simulink model "testSerializedParams"  (R2014a)
settings: Solver=FixedStepDiscrete  StartTime=0.0  StopTime=Inf  FixedStep=0.001  RelTol=1e-3
InitFcn:
  | testSerializedParams_Initialize();
undefined symbols (not defined in the file or in its folder): fn5, libBusSerialize, TestBus_serializedParam
libraries: slrtlib x5, dspswit3 x2, libButtons x1
settings Model: BufferReuse=off  Creator=shenoylab  LastModifiedBy=djoshea
settings SolverCC: EnableConcurrentExecution=on
settings DataIOCC: SignalLoggingSaveFormat=ModelDataLogs
settings OptimizationCC: BlockReduction=off  OptimizeBlockIOStorage=off  BufferReuse=off  GlobalBufferReuse=off  ExpressionFolding=off  LocalBlockOutputs=off
settings DebuggingCC: MultiTaskDSMMsg=warning  MultiTaskCondExecSysMsg=none  StateNameClashWarn=warning
settings HardwareCC: ProdIntDivRoundTo=Zero  ProdEndianess=LittleEndian  ProdHWDeviceType=Generic->32-bit x86 compatible
settings RTWCC: SystemTargetFile=slrt.tlc  TemplateMakefile=slrt_default_tmf  Description=Simulink Real-Time  GenerateReport=on  ProcessScript=slrt_make_rtw_hook  LaunchReport=on  IncludeERTFirstTime=on  RTWCompilerOptimization=On
settings CodeAppCC: MATLABSourceComments=on
settings SimulinkRealTimeCC: GeneratePreprocessorConditionals=Disable all  EnableShiftOperators=on

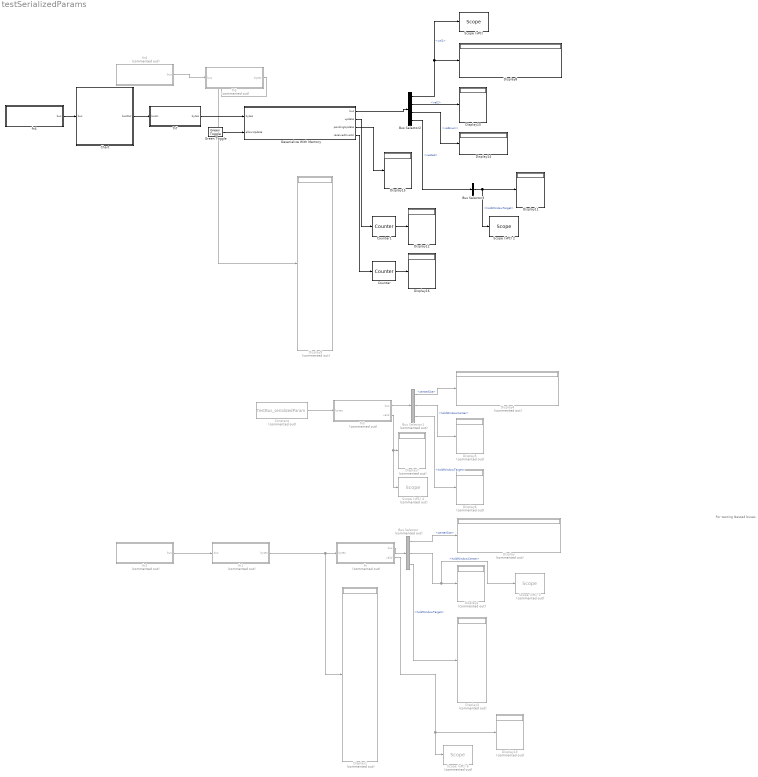
== system testSerializedParams ==
  note: For testing Nested buses
  Bus Selector : BusSelector  Commented=on  OutputSignals=centerSize,holdWindowCenter,holdWindowTarget
  Bus Selector1 : BusSelector  Commented=on  OutputSignals=centerSize,holdWindowCenter,holdWindowTarget
  Bus Selector2 : BusSelector  OutputSignals=val1,val2,valEnum,nested
  Bus Selector3 : BusSelector  OutputSignals=holdWindowTarget
  Chart : Stateflow chart  TreatAsAtomicUnit=on
  Constant : Constant  Commented=on  Value=TestBus_serializedParam  OutDataTypeStr=uint8
  Counter : dspswit3/Counter  Direction=Up  CountEvent=Non-zero sample  CounterSize=32 bits  MaxCount=255  InitialCount=0  Output=Count  HitValue=32  ResetInput=off  SamplesPerFrame=1  Ts=1  CntDtype=uint32  HitDtype=Logical
  Counter1 : dspswit3/Counter  Direction=Up  CountEvent=Non-zero sample  CounterSize=32 bits  MaxCount=255  InitialCount=0  Output=Count  HitValue=32  ResetInput=off  SamplesPerFrame=1  Ts=1  CntDtype=uint32  HitDtype=Logical
  Deserialize With Memory : MATLAB Function  TreatAsAtomicUnit=on  mask(Deserialize Bus With Internal Memory){busType=Bus: TestBusOuter}
      mask prompts: busType "Bus Type:"
      mask help:
      | This block deserializes a uint8 bytestream into a specific bus type. When the input changes, the block will deserialize the new input, and the deserialization is successful, it will internally store the updated bus.
      |
      | If allowUpdate is high at that point, the new bus value will be output immediately and update will be driven high. If not, pendingUpdate will be driven high, and the updated bus will be held in an internal persistent variable. When allowUpdate goes high, this updated bus will be passed to the output, and update will be driven high.
      |
      | If an invalid serialized bus is received, receivedInvalid will be driven high, and the bus output will not change from its previously stored value. If the initial value sent to this block is invalid, a default initialized bus will be output with all zeros or empty bus elements.
      mask init:
      | BusSerialize.maskDeserializeMemoryBlockUpdate(gcb);
  Display{,1..7,9,13} (10 alike) : Display  Commented=on
  Display{8,10..12,14..16} (7 alike) : Display
  Green Toggle : libButtons/Green Toggle  SystemSampleTime=-1
  "Scope (xPC) " : slrtlib/Displays and Logging/Scope   scopeno=1  scopetype=Target  autostart=on  viewmode=Numerical  formatstr='%15.6f'  grid=on  ylimits=[0,0]  nosamples=250  noprepostsamples=0  interleave=1  triggermode=FreeRun  triggersignal=1  trigsignalfromport=off  triggerlevel=0.0  triggerslope=Either  triggerscope=1  triggersample=0  filename=data.dat  mode=Lazy  writesize=512  autorestart=off  dynamicfilemode=off  maxwritefilesize=512*1024^2
  Scope (xPC) 2 : slrtlib/Displays and Logging/Scope   scopeno=3  scopetype=Target  autostart=on  viewmode=Numerical  formatstr='%15.6f'  grid=on  ylimits=[0,0]  nosamples=250  noprepostsamples=0  interleave=1  triggermode=FreeRun  triggersignal=1  trigsignalfromport=off  triggerlevel=0.0  triggerslope=Either  triggerscope=1  triggersample=0  filename=data.dat  mode=Lazy  writesize=512  autorestart=off  dynamicfilemode=off  maxwritefilesize=512*1024^2
  Scope (xPC) 3 : slrtlib/Displays and Logging/Scope   Commented=on  scopeno=4  scopetype=Target  autostart=on  viewmode=Numerical  formatstr='%15.6f'  grid=on  ylimits=[0,0]  nosamples=250  noprepostsamples=0  interleave=1  triggermode=FreeRun  triggersignal=1  trigsignalfromport=off  triggerlevel=0.0  triggerslope=Either  triggerscope=1  triggersample=0  filename=data.dat  mode=Lazy  writesize=512  autorestart=off  dynamicfilemode=off  maxwritefilesize=512*1024^2
  Scope (xPC) 4 : slrtlib/Displays and Logging/Scope   Commented=on  scopeno=5  scopetype=Target  autostart=on  viewmode=Numerical  formatstr='%15.6f'  grid=on  ylimits=[0,0]  nosamples=250  noprepostsamples=0  interleave=1  triggermode=FreeRun  triggersignal=1  trigsignalfromport=off  triggerlevel=0.0  triggerslope=Either  triggerscope=1  triggersample=0  filename=data.dat  mode=Lazy  writesize=512  autorestart=off  dynamicfilemode=off  maxwritefilesize=512*1024^2
  Scope (xPC) 6 : slrtlib/Displays and Logging/Scope   Commented=on  scopeno=6  scopetype=Target  autostart=on  viewmode=Numerical  formatstr='%15.6f'  grid=on  ylimits=[0,0]  nosamples=250  noprepostsamples=0  interleave=1  triggermode=FreeRun  triggersignal=1  trigsignalfromport=off  triggerlevel=0.0  triggerslope=Either  triggerscope=1  triggersample=0  filename=data.dat  mode=Lazy  writesize=512  autorestart=off  dynamicfilemode=off  maxwritefilesize=512*1024^2
  fn : MATLAB Function  Commented=on  TreatAsAtomicUnit=on
  fn1 : MATLAB Function  Commented=on  TreatAsAtomicUnit=on
  fn2 : MATLAB Function  Commented=on  TreatAsAtomicUnit=on
  fn3 : MATLAB Function  Commented=on  TreatAsAtomicUnit=on
  fn4 : MATLAB Function  TreatAsAtomicUnit=on
  fn5 : MATLAB Function  Commented=on  TreatAsAtomicUnit=on
  fn6 : MATLAB Function  Commented=on  TreatAsAtomicUnit=on
  fn7 : MATLAB Function  AncestorBlock=libBusSerialize/fn5  TreatAsAtomicUnit=on  mask(BusSerialize: serialize block){busType=Bus: TestBusOuter}
      mask prompts: busType "Bus Type"
      mask help: Select the bus type below to serialize.
      mask init:
      | BusSerialize.maskSerializeBlockUpdate(gcb)
  wires:
  fn/1(bus) -> Bus Selector/1
  fn1/1(bytes) -> Display1/1, fn/1(bytes)
  fn2/1(bus) -> fn1/1(bus)
  Bus Selector/1 -> Display/1  "<centerSize>"
  Bus Selector/2 -> Scope (xPC) 3/1, Display2/1  "<holdWindowCenter>"
  Bus Selector/3 -> Display3/1  "<holdWindowTarget>"
  Constant/1 -> fn3/1(bytes)
  Bus Selector1/1 -> Display4/1  "<centerSize>"
  Bus Selector1/2 -> Display5/1  "<holdWindowCenter>"
  Bus Selector1/3 -> Display6/1  "<holdWindowTarget>"
  fn3/1(bus) -> Bus Selector1/1
  fn3/2(valid) -> Scope (xPC) 4/1, Display7/1
  Bus Selector2/1 -> "Scope (xPC) "/1, Display8/1  "<val1>"
  Bus Selector2/2 -> Display10/1  "<val2>"
  Bus Selector2/4 -> Bus Selector3/1  "<nested>"
  Bus Selector3/1 -> Scope (xPC) 2/1, Display11/1  "<holdWindowTarget>"
  fn/2(valid) -> Scope (xPC) 6/1, Display13/1
  Bus Selector2/3 -> Display14/1  "<valEnum>"
  fn5/1(bytes) -> Display9/1
  fn6/1(bus) -> fn5/1(bus)
  Deserialize With Memory/1(bus) -> Bus Selector2/1
  fn7/1(bytes) -> Deserialize With Memory/1(bytes)
  Deserialize With Memory/3(pendingUpdate) -> Display15/1
  Deserialize With Memory/4(receivedInvalid) -> Counter/1
  Counter/1 -> Display16/1
  Deserialize With Memory/2(update) -> Counter1/1
  Counter1/1 -> Display12/1
  Green Toggle/1 -> Deserialize With Memory/2(allowUpdate)
  fn4/1(bus) -> Chart/1(bus)
  Chart/1(busOut) -> fn7/1(busIn)

== matlab function testSerializedParams/fn1 ==
  data: bus input Bus: TestBus size=1; bytes output uint8 size=200
function bytes = serialize(bus)
%#codegen

bytes = testSerializedParamsLib.serializeBus_TestBus(bus);

== matlab function testSerializedParams/fn ==
  data: bytes input uint8; bus output Bus: TestBus; valid output uint8 size=1
function [bus, valid] = deserialize(bytes)
%#codegen

[bus, valid] = testSerializedParamsLib.deserializeBus_TestBus(bytes);

== matlab function testSerializedParams/fn2 ==
  data: bus output Bus: TestBus size=1
function bus = createBus()

coder.varsize('bus.centerSize', [3 3]);
coder.varsize('bus.holdWindowTarget', 30);
bus.centerSize = uint16([1 2; 3 4]);
bus.holdWindowCenter = uint8(15);
bus.holdWindowTarget = uint8('hello world')';

== matlab function testSerializedParams/fn3 ==
  data: bytes input uint8; bus output Bus: TestBus; valid output uint8 size=1
function [bus, valid] = deserialize(bytes)
%#codegen

[bus, valid] = testSerializedParamsLib.deserializeBus_TestBus(bytes);

== matlab function testSerializedParams/Deserialize With Memory ==
  data: bytes input uint8; bus output Bus: TestBusOuter size=1; allowUpdate input uint8 size=1; update output uint8 size=1; pendingUpdate output uint8 size=1; receivedInvalid output uint8 size=1
function [bus, update, pendingUpdate, receivedInvalid] = deserializeWithMemory(bytes, allowUpdate)

%#codegen



    % cache input so we only deserialize on changes

    persistent pBytes;

    if isempty(pBytes)

        pBytes = bytes;

        inChanged = uint8(1);

    elseif ~isequal(pBytes, bytes)

        pBytes = bytes;

        inChanged = uint8(1);

    else

        inChanged = uint8(0);

    end



    % internal most up to date input received

    persistent pBusLatest;

    if isempty(pBusLatest)

        pBusLatest =  testSerializedParamsLib.initializeBus_TestBusOuter();

    end



    % external cached output

    persistent pBusOut;

    if isempty(pBusOut)

        pBusOut = pBusLatest;

    end



    % is an update pending allowUpdate == 1?

    persistent pPendingUpdate

    if isempty(pPendingUpdate)

        pPendingUpdate = uint8(0);

    end



    % handle deserialization if changed

    receivedUpdate = uint8(0);

    receivedInvalid = uint8(0);

    if inChanged

        [tempBus, valid] = testSerializedParamsLib.deserializeBus_TestBusOuter(bytes);

        if valid

            pBusLatest = tempBus;

            receivedUpdate = uint8(1);

            pPendingUpdate = uint8(1);

        else

            receivedInvalid = uint8(1);

        end

    end

    

    update = uint8(0);

    pendingUpdate = uint8(0);

    

    % handle internal buffering

    if pPendingUpdate

        if allowUpdate

            % pass the updated bus out

            pBusOut = pBusLatest;

            update = uint8(1);

            pendingUpdate = uint8(0);

            pPendingUpdate = uint8(0); % no longer pending

        else

            % hold the updated bus internally for now

            update = uint8(0);

            pendingUpdate = uint8(1);

        end

    else

        update = uint8(0);

        pendingUpdate = uint8(0);

    end

         

    bus = pBusOut;

    

end

== matlab function testSerializedParams/fn5 ==
  data: bus input Bus: TestBusOuter size=1; bytes output uint8 size=300
function bytes = serialize(bus)
%#codegen

bytes = testSerializedParamsLib.serializeBus_TestBusOuter(bus);

== matlab function testSerializedParams/fn6 ==
  data: bus output Bus: TestBusOuter size=1
function bus = createBus()

bus = testSerializedParamsLib.initializeBus_TestBusOuter();
P1 = testSerializedParamsLib.initializeBus_TestBusInner();

P1.centerSize = uint8([1 2])';
P1.holdWindowCenter = uint8(2);
P1.holdWindowTarget = uint16(30);

bus.val1 = uint8(3);
bus.val2 = uint8('hello')';
bus.valEnum = TestEnum.eval3_longer;
bus.nested = P1;

== matlab function testSerializedParams/fn4 ==
  data: bus output Bus: TestBusOuter size=1
function bus = createBus()

bus = testSerializedParamsLib.initializeBus_TestBusOuter();
P1 = testSerializedParamsLib.initializeBus_TestBusInner();

P1.centerSize = uint8([1 2])';
P1.holdWindowCenter = uint8(2);
P1.holdWindowTarget = uint16(30);

bus.val1 = uint8(3);
bus.val2 = uint8('hello')';
bus.valEnum = TestEnum.eval3_longer;
bus.nested = P1;

== stateflow chart testSerializedParams/Chart ==
  state s1
    du:
    busOut = bus;
    busOut.valEnum = TestEnum.eval2;
  state s2
    du:
    busOut = bus;
    busOut.valEnum = TestEnum.eval3_longer;
  (default) -> s1
  s2 -> s1 : after(5000,tick)
  s1 -> s2 : after(5000, tick)
  data: bus input Bus: TestBusOuter; busOut output Bus: TestBusOuter

== matlab function testSerializedParams/fn7 ==
  data: busIn input Bus: TestBusOuter size=1; bytes output uint8 size=162
function bytes = serialize(busIn)
%#codegen, 

    coder.varsize('pBytes', 162);
    coder.varsize('bytes', 162);

    persistent pBus;
    persistent pBytes;
    if isempty(pBus)
        pBus = busIn;
        pBytes = zeros(0, 1, 'uint8');
        changed = uint8(1);
        
    elseif ~isequal(pBus, busIn)
        pBus = busIn;
        changed = uint8(1);
    else
        changed = uint8(0);
    end

    if changed
        pBytes = testSerializedParamsLib.serializeBus_TestBusOuter(busIn);
    end
    
    bytes = pBytes;
end
